simulink model "E_Toothbrush_05"  (Simulink 7.8)
settings: Solver=ode3  StartTime=0.0  StopTime=20  FixedStep=0.001  RelTol=1e-3
undefined symbols (not defined in the file or in its folder): Bar1_length, Bar3_end_xyz, Bar4_length, Body_inertia, Body_mass, Load_torque, Main_gear_r, Motor_gear_r, Motor_speed, Stall_torque
libraries: mblibv1 x31, simulink x1
settings Model: Creator=Harvey  LastModifiedBy=Harvey
settings SimMechanicsCC: VisOnUpdateDiagram=on  VisDuringSimulation=on

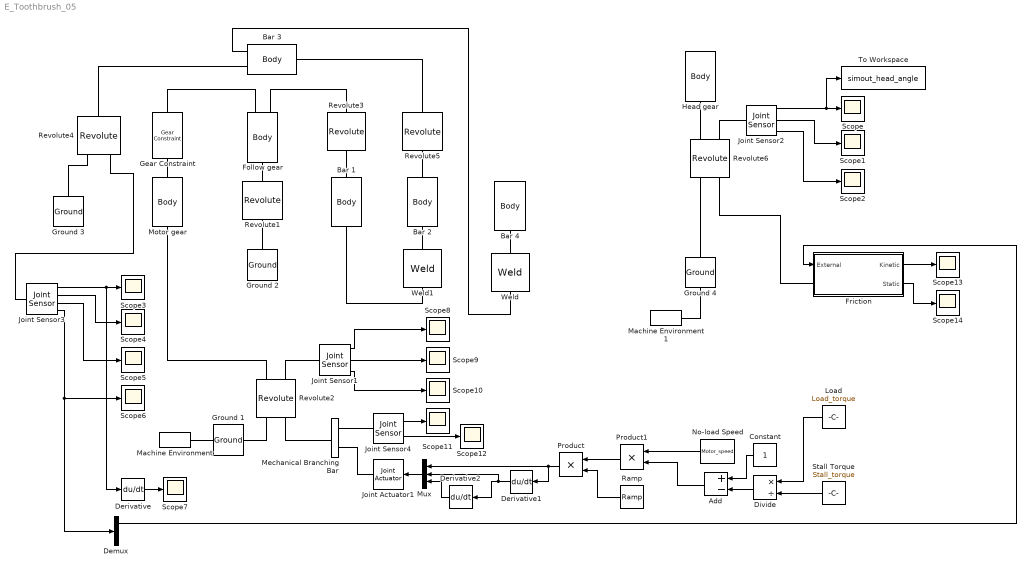
== system E_Toothbrush_05 ==
  Add : Sum  Inputs=+-
  Bar 1 : mblibv1/Bodies/Body  LConnTagsString=CS1  RConnTagsString=CS2  UpdateFromCAD=off  DialogClass=MechanicalBodyBlock  Mass=Body_mass  MassUnits=g  InertiaUnits=g*cm^2  Inertia=Body_inertia  Shape=Cylinder  ShapeDims=[1 1]  ShapeUnits=m  ShapeUse=false  Density=1  DensityUnits=kg/m^3  DensityUse=false  GraphicsMode=MACHINE_DEFAULT  BodyColorSelMode=COLORPALETTE  BodyColor=[0.87059 0.4902 0]  AttachedToCS=CG  CG=Left$CG$[0 0 Bar1_length/2]$CS1$CS1$mm$[0 0 0]$Euler X-Y-Z$deg$WORLD$false$none  WorkingFrames=Left$CS1$[0 0 0]$Adjoining$Adjoining$mm$[0 0 0]$Euler X-Y-Z$deg$WORLD$true$none#Right$CS2$[0 0 Bar1_length]$CS1$CS1$mm$[0 0 0]$Euler X-Y-Z$deg$WORLD$true$none  CGPos=[0 0 Bar1_length/2]  CGRot=[0 0 0]  CS0Pos=[]  CS0Rot=[]  CS1Pos=[0 0 0]  CS1Rot=[0 0 0]  CS2Pos=[0 0 Bar1_length]  CS2Rot=[0 0 0]  CS3Pos=[]  CS3Rot=[]  CS4Pos=[]  CS4Rot=[]  CS5Pos=[]  CS5Rot=[]  CS6Pos=[]  CS6Rot=[]  CS7Pos=[]  CS7Rot=[]  CS8Pos=[]  CS8Rot=[]  CS9Pos=[]  CS9Rot=[]  CS10Pos=[]  CS10Rot=[]  CS11Pos=[]  CS11Rot=[]  CS12Pos=[]  CS12Rot=[]  CS13Pos=[]  CS13Rot=[]  CS14Pos=[]  CS14Rot=[]  CS15Pos=[]  CS15Rot=[]  CS16Pos=[]  CS16Rot=[]  CS17Pos=[]  CS17Rot=[]  CS18Pos=[]  CS18Rot=[]  CS19Pos=[]  CS19Rot=[]  CS20Pos=[]  CS20Rot=[]
  Bar 2 : mblibv1/Bodies/Body  LConnTagsString=CS1  RConnTagsString=CS2  UpdateFromCAD=off  DialogClass=MechanicalBodyBlock  Mass=Body_mass  MassUnits=g  InertiaUnits=g*cm^2  Inertia=Body_inertia  Shape=Cylinder  ShapeDims=[1 1]  ShapeUnits=m  ShapeUse=false  Density=1  DensityUnits=kg/m^3  DensityUse=false  GraphicsMode=MACHINE_DEFAULT  BodyColorSelMode=COLORPALETTE  BodyColor=[0 0 1]  AttachedToCS=CG  CG=Left$CG$[0 0 0]$CS1$CS1$mm$[0 0 0]$Euler X-Y-Z$deg$WORLD$false$none  WorkingFrames=Left$CS1$[0 0 0]$Adjoining$Adjoining$mm$[0 0 0]$Euler X-Y-Z$deg$WORLD$true$none#Right$CS2$[0 0 0]$Adjoining$Adjoining$mm$[0 0 0]$Euler X-Y-Z$deg$WORLD$true$none  CGPos=[0 0 0]  CGRot=[0 0 0]  CS0Pos=[]  CS0Rot=[]  CS1Pos=[0 0 0]  CS1Rot=[0 0 0]  CS2Pos=[0 0 0]  CS2Rot=[0 0 0]  CS3Pos=[]  CS3Rot=[]  CS4Pos=[]  CS4Rot=[]  CS5Pos=[]  CS5Rot=[]  CS6Pos=[]  CS6Rot=[]  CS7Pos=[]  CS7Rot=[]  CS8Pos=[]  CS8Rot=[]  CS9Pos=[]  CS9Rot=[]  CS10Pos=[]  CS10Rot=[]  CS11Pos=[]  CS11Rot=[]  CS12Pos=[]  CS12Rot=[]  CS13Pos=[]  CS13Rot=[]  CS14Pos=[]  CS14Rot=[]  CS15Pos=[]  CS15Rot=[]  CS16Pos=[]  CS16Rot=[]  CS17Pos=[]  CS17Rot=[]  CS18Pos=[]  CS18Rot=[]  CS19Pos=[]  CS19Rot=[]  CS20Pos=[]  CS20Rot=[]
  Bar 3 : mblibv1/Bodies/Body  LConnTagsString=CS2  RConnTagsString=CS3|CS1  UpdateFromCAD=off  DialogClass=MechanicalBodyBlock  Mass=Body_mass  MassUnits=g  InertiaUnits=g*cm^2  Inertia=Body_inertia  Shape=Cylinder  ShapeDims=[1 1]  ShapeUnits=m  ShapeUse=false  Density=1  DensityUnits=kg/m^3  DensityUse=false  GraphicsMode=MACHINE_DEFAULT  BodyColorSelMode=COLORPALETTE  BodyColor=[0 1 0]  AttachedToCS=CG  CG=Left$CG$Bar3_end_xyz/2$CS1$CS1$mm$[0 0 0]$Euler X-Y-Z$deg$WORLD$false$none  WorkingFrames=Right$CS3$[0 0 0]$CS1$CS1$mm$[0 0 0]$Euler X-Y-Z$deg$WORLD$true$none#Right$CS1$[0 0 0]$Adjoining$Adjoining$mm$[0 0 0]$Euler X-Y-Z$deg$WORLD$true$none#Left$CS2$Bar3_end_xyz$CS1$CS1$mm$[0 0 0]$Euler X-Y-Z$deg$WORLD$true$none  CGPos=Bar3_end_xyz/2  CGRot=[0 0 0]  CS0Pos=[]  CS0Rot=[]  CS1Pos=[0 0 0]  CS1Rot=[0 0 0]  CS2Pos=Bar3_end_xyz  CS2Rot=[0 0 0]  CS3Pos=[0 0 0]  CS3Rot=[0 0 0]  CS4Pos=[]  CS4Rot=[]  CS5Pos=[]  CS5Rot=[]  CS6Pos=[]  CS6Rot=[]  CS7Pos=[]  CS7Rot=[]  CS8Pos=[]  CS8Rot=[]  CS9Pos=[]  CS9Rot=[]  CS10Pos=[]  CS10Rot=[]  CS11Pos=[]  CS11Rot=[]  CS12Pos=[]  CS12Rot=[]  CS13Pos=[]  CS13Rot=[]  CS14Pos=[]  CS14Rot=[]  CS15Pos=[]  CS15Rot=[]  CS16Pos=[]  CS16Rot=[]  CS17Pos=[]  CS17Rot=[]  CS18Pos=[]  CS18Rot=[]  CS19Pos=[]  CS19Rot=[]  CS20Pos=[]  CS20Rot=[]
  Bar 4 : mblibv1/Bodies/Body  LConnTagsString=CS1  RConnTagsString=CS2  UpdateFromCAD=off  DialogClass=MechanicalBodyBlock  Mass=Body_mass  MassUnits=g  InertiaUnits=g*cm^2  Inertia=Body_inertia  Shape=Cylinder  ShapeDims=[1 1]  ShapeUnits=m  ShapeUse=false  Density=1  DensityUnits=kg/m^3  DensityUse=false  GraphicsMode=MACHINE_DEFAULT  BodyColorSelMode=COLORPALETTE  BodyColor=[1 1 0]  AttachedToCS=CG  CG=Left$CG$[0 0 Bar4_length/2]$CS1$CS1$mm$[0 0 0]$Euler X-Y-Z$deg$WORLD$false$none  WorkingFrames=Left$CS1$[0 0 0]$Adjoining$Adjoining$mm$[0 0 0]$Euler X-Y-Z$deg$WORLD$true$none#Right$CS2$[0 0 Bar4_length]$CS1$CS1$mm$[0 0 0]$Euler X-Y-Z$deg$WORLD$true$none  CGPos=[0 0 Bar4_length/2]  CGRot=[0 0 0]  CS0Pos=[]  CS0Rot=[]  CS1Pos=[0 0 0]  CS1Rot=[0 0 0]  CS2Pos=[0 0 Bar4_length]  CS2Rot=[0 0 0]  CS3Pos=[]  CS3Rot=[]  CS4Pos=[]  CS4Rot=[]  CS5Pos=[]  CS5Rot=[]  CS6Pos=[]  CS6Rot=[]  CS7Pos=[]  CS7Rot=[]  CS8Pos=[]  CS8Rot=[]  CS9Pos=[]  CS9Rot=[]  CS10Pos=[]  CS10Rot=[]  CS11Pos=[]  CS11Rot=[]  CS12Pos=[]  CS12Rot=[]  CS13Pos=[]  CS13Rot=[]  CS14Pos=[]  CS14Rot=[]  CS15Pos=[]  CS15Rot=[]  CS16Pos=[]  CS16Rot=[]  CS17Pos=[]  CS17Rot=[]  CS18Pos=[]  CS18Rot=[]  CS19Pos=[]  CS19Rot=[]  CS20Pos=[]  CS20Rot=[]
  Constant : Constant
  Demux : Demux  Outputs=3
  Derivative : Derivative
  Derivative1 : Derivative
  Derivative2 : Derivative
  Divide : Product  Inputs=*/
  Follow gear : mblibv1/Bodies/Body  LConnTagsString=CS1  RConnTagsString=CS2|CS3  UpdateFromCAD=off  DialogClass=MechanicalBodyBlock  Mass=Body_mass  MassUnits=g  InertiaUnits=g*cm^2  Inertia=Body_inertia  Shape=Cylinder  ShapeDims=[1 1]  ShapeUnits=m  ShapeUse=false  Density=1  DensityUnits=kg/m^3  DensityUse=false  GraphicsMode=MACHINE_DEFAULT  BodyColorSelMode=COLORPALETTE  BodyColor=[1 0.6 0.78431]  AttachedToCS=CG  CG=Left$CG$[0 0 0]$CS1$CS1$mm$[0 0 0]$Euler X-Y-Z$deg$WORLD$false$none  WorkingFrames=Left$CS1$[0 0 0]$Adjoining$Adjoining$mm$[0 0 0]$Euler X-Y-Z$deg$WORLD$true$none#Right$CS2$[0 0 0]$CS1$CS1$mm$[0 0 0]$Euler X-Y-Z$deg$WORLD$true$none#Right$CS3$Bar1_start_xyz$World$World$mm$[0 0 0]$Euler X-Y-Z$deg$WORLD$true$none  CGPos=[0 0 0]  CGRot=[0 0 0]  CS0Pos=[]  CS0Rot=[]  CS1Pos=[0 0 0]  CS1Rot=[0 0 0]  CS2Pos=[0 0 0]  CS2Rot=[0 0 0]  CS3Pos=Bar1_start_xyz  CS3Rot=[0 0 0]  CS4Pos=[]  CS4Rot=[]  CS5Pos=[]  CS5Rot=[]  CS6Pos=[]  CS6Rot=[]  CS7Pos=[]  CS7Rot=[]  CS8Pos=[]  CS8Rot=[]  CS9Pos=[]  CS9Rot=[]  CS10Pos=[]  CS10Rot=[]  CS11Pos=[]  CS11Rot=[]  CS12Pos=[]  CS12Rot=[]  CS13Pos=[]  CS13Rot=[]  CS14Pos=[]  CS14Rot=[]  CS15Pos=[]  CS15Rot=[]  CS16Pos=[]  CS16Rot=[]  CS17Pos=[]  CS17Rot=[]  CS18Pos=[]  CS18Rot=[]  CS19Pos=[]  CS19Rot=[]  CS20Pos=[]  CS20Rot=[]
  Friction : Subsystem
  Gear Constraint : mblibv1/Constraints &  Drivers/Gear Constraint  LConnTagsString=__newl0  RConnTagsString=__newr0  UpdateFromCAD=off  DialogClass=GearConstraint  NumSAPorts=0  BaseRadius=Motor_gear_r  BaseRadiusUnits=mm  FollowerRadius=Main_gear_r  FollowerRadiusUnits=mm
  Ground 1 : mblibv1/Bodies/Ground  UpdateFromCAD=off  LeftPortType=env  RightPortType=workingframe  PhysicalDomain=Mechanical  DialogClass=GroundBlock  CoordPosition=[0 0 0]  CoordPositionUnits=mm  StateVectorMgrId=2  MachineId=[1 1]  ShowEnvPort=on
  Ground 2 : mblibv1/Bodies/Ground  UpdateFromCAD=off  LeftPortType=env  RightPortType=workingframe  PhysicalDomain=Mechanical  DialogClass=GroundBlock  CoordPosition=[Motor_gear_r+Main_gear_r 0 0]  CoordPositionUnits=mm  StateVectorMgrId=-1  MachineId=[0 0]  ShowEnvPort=off
  Ground 3 : mblibv1/Bodies/Ground  UpdateFromCAD=off  LeftPortType=env  RightPortType=workingframe  PhysicalDomain=Mechanical  DialogClass=GroundBlock  CoordPosition=[0 0 Bar1_length]  CoordPositionUnits=mm  StateVectorMgrId=-1  MachineId=[0 0]  ShowEnvPort=off
  Ground 4 : mblibv1/Bodies/Ground  UpdateFromCAD=off  LeftPortType=env  RightPortType=workingframe  PhysicalDomain=Mechanical  DialogClass=GroundBlock  CoordPosition=Head_xyz  CoordPositionUnits=mm  StateVectorMgrId=3  MachineId=[1 0]  ShowEnvPort=on
  Head gear : mblibv1/Bodies/Body  LConnTagsString=CS1  RConnTagsString=CS2  UpdateFromCAD=off  DialogClass=MechanicalBodyBlock  Mass=1  MassUnits=g  InertiaUnits=g*cm^2  Inertia=Body_inertia  Shape=Cylinder  ShapeDims=[1 1]  ShapeUnits=m  ShapeUse=false  Density=1  DensityUnits=kg/m^3  DensityUse=false  GraphicsMode=MACHINE_DEFAULT  BodyColorSelMode=COLORPALETTE  BodyColor=[0.47843 0.062745 0.89412]  AttachedToCS=CG  CG=Left$CG$[0 0 0]$CS1$CS1$mm$[0 0 0]$Euler X-Y-Z$deg$CS1$false$none  WorkingFrames=Left$CS1$[0 0 0]$Adjoining$Adjoining$mm$[0 0 0]$Euler X-Y-Z$deg$World$true$none#Right$CS2$[0 5 0]$CS1$CS1$mm$[0 0 0]$Euler X-Y-Z$deg$CS1$true$none#Right$CS3$[0 -5 0]$CS1$CS1$mm$[0 0 0]$Euler X-Y-Z$deg$CS1$false$none  CGPos=[0 0 0]  CGRot=[0 0 0]  CS0Pos=[]  CS0Rot=[]  CS1Pos=[0 0 0]  CS1Rot=[0 0 0]  CS2Pos=[0 5 0]  CS2Rot=[0 0 0]  CS3Pos=[0 -5 0]  CS3Rot=[0 0 0]  CS4Pos=[]  CS4Rot=[]  CS5Pos=[]  CS5Rot=[]  CS6Pos=[]  CS6Rot=[]  CS7Pos=[]  CS7Rot=[]  CS8Pos=[]  CS8Rot=[]  CS9Pos=[]  CS9Rot=[]  CS10Pos=[]  CS10Rot=[]  CS11Pos=[]  CS11Rot=[]  CS12Pos=[]  CS12Rot=[]  CS13Pos=[]  CS13Rot=[]  CS14Pos=[]  CS14Rot=[]  CS15Pos=[]  CS15Rot=[]  CS16Pos=[]  CS16Rot=[]  CS17Pos=[]  CS17Rot=[]  CS18Pos=[]  CS18Rot=[]  CS19Pos=[]  CS19Rot=[]  CS20Pos=[]  CS20Rot=[]
  Joint Actuator1 : mblibv1/Sensors &  Actuators/Joint Actuator  UpdateFromCAD=off  PhysicalDomain=Mechanical  PortType=blob  ActuationStyle=Motion  AngleUnits=deg  ArcVelocityUnits=rpm  ArcAccelerationUnits=deg/s^2  CoordPositionUnits=m  VelocityUnits=m/s  AccelerationUnits=m/s^2  ForceUnits=N  TorqueUnits=mN*m  ActiveIO=on  Width=3  DialogClass=MechanicalActuatorBlock  Primitive=R1  ReferenceFrame=Absolute (World)
  Joint Sensor1 : mblibv1/Sensors &  Actuators/Joint Sensor  UpdateFromCAD=off  PhysicalDomain=Mechanical  PortType=blob  Muxed=off  Pose=off  Angle=on  AngleUnits=deg  ArcVelocity=on  ArcVelocityUnits=rpm  ArcAcceleration=off  ArcAccelerationUnits=deg/s^2  CoordPosition=on  CoordPositionUnits=m  Velocity=off  VelocityUnits=m/s  Acceleration=off  AccelerationUnits=m/s^2  Quaternion=on  QuaternionDT=off  QuaternionDDT=off  QuaternionUnits=off  OutputVector=[1]  ActiveIO=on  Width=3  DialogClass=MechanicalSensorBlock  Primitive=R1  Force=off  ForceUnits=N  Torque=on  TorqueUnits=N*m  ReferenceFrame=Absolute (World)  ReactionSensedSide=Follower  ReactionReferenceFrame=Local (Body CS)  ReactionForce=off  ReactionForceUnits=N  ReactionMoment=off  ReactionMomentUnits=N*m
  Joint Sensor2 : mblibv1/Sensors &  Actuators/Joint Sensor  UpdateFromCAD=off  PhysicalDomain=Mechanical  PortType=blob  Muxed=off  Pose=off  Angle=on  AngleUnits=deg  ArcVelocity=on  ArcVelocityUnits=rpm  ArcAcceleration=off  ArcAccelerationUnits=deg/s^2  CoordPosition=on  CoordPositionUnits=m  Velocity=off  VelocityUnits=m/s  Acceleration=off  AccelerationUnits=m/s^2  Quaternion=on  QuaternionDT=off  QuaternionDDT=off  QuaternionUnits=off  OutputVector=[1]  ActiveIO=on  Width=5  DialogClass=MechanicalSensorBlock  Primitive=R1  Force=off  ForceUnits=N  Torque=off  TorqueUnits=N*m  ReferenceFrame=Absolute (World)  ReactionSensedSide=Base  ReactionReferenceFrame=Absolute (World)  ReactionForce=off  ReactionForceUnits=N  ReactionMoment=on  ReactionMomentUnits=N*m
  Joint Sensor3 : mblibv1/Sensors &  Actuators/Joint Sensor  UpdateFromCAD=off  PhysicalDomain=Mechanical  PortType=blob  Muxed=off  Pose=off  Angle=on  AngleUnits=deg  ArcVelocity=on  ArcVelocityUnits=rpm  ArcAcceleration=on  ArcAccelerationUnits=deg/s^2  CoordPosition=on  CoordPositionUnits=m  Velocity=off  VelocityUnits=m/s  Acceleration=off  AccelerationUnits=m/s^2  Quaternion=on  QuaternionDT=off  QuaternionDDT=off  QuaternionUnits=off  OutputVector=[1]  ActiveIO=on  Width=6  DialogClass=MechanicalSensorBlock  Primitive=R1  Force=off  ForceUnits=N  Torque=off  TorqueUnits=N*m  ReferenceFrame=Absolute (World)  ReactionSensedSide=Follower  ReactionReferenceFrame=Absolute (World)  ReactionForce=off  ReactionForceUnits=N  ReactionMoment=on  ReactionMomentUnits=N*m
  Joint Sensor4 : mblibv1/Sensors &  Actuators/Joint Sensor  UpdateFromCAD=off  PhysicalDomain=Mechanical  PortType=blob  Muxed=off  Pose=off  Angle=on  AngleUnits=deg  ArcVelocity=on  ArcVelocityUnits=rpm  ArcAcceleration=off  ArcAccelerationUnits=deg/s^2  CoordPosition=on  CoordPositionUnits=m  Velocity=off  VelocityUnits=m/s  Acceleration=off  AccelerationUnits=m/s^2  Quaternion=on  QuaternionDT=off  QuaternionDDT=off  QuaternionUnits=off  OutputVector=[1]  ActiveIO=on  Width=2  DialogClass=MechanicalSensorBlock  Primitive=R1  Force=off  ForceUnits=N  Torque=off  TorqueUnits=N*m  ReferenceFrame=Absolute (World)  ReactionSensedSide=Base  ReactionReferenceFrame=Absolute (World)  ReactionForce=off  ReactionForceUnits=N  ReactionMoment=off  ReactionMomentUnits=N*m
  Load : Constant  Value=Load_torque
  Machine Environment : mblibv1/Bodies/Machine Environment  PortType=env  PhysicalDomain=Mechanical  DialogTemplateClass=MECH.MachineEnvironment  SyncWhenCopied=off  Gravity=[0 0 -9.81]  GravityUnits=m/s^2  GravityAsSignal=off  Dimensionality=3D Only  AnalysisType=Forward dynamics  LinearAssemblyTolerance=1e-3  LinearAssemblyToleranceUnits=m  AngularAssemblyTolerance=1e-3  AngularAssemblyToleranceUnits=rad  ConstraintSolverType=Stabilizing  ConstraintRelTolerance=1e-4  ConstraintAbsTolerance=1e-4  UseRobustSingularityHandling=off  RedundancyAnalysisToleranceType=Automatically select tolerance  RedundancyAnalysisTolerance=1e-14  StatePerturbationType=Fixed  PerturbationSize=1e-5  VisualizeMachine=on  BodyVisualizationType=Use model default body geometries  BodyColorSelMode=Use model default  DefaultBodyColor=[1 0 0]
  Machine Environment1 : mblibv1/Bodies/Machine Environment  PortType=env  PhysicalDomain=Mechanical  DialogTemplateClass=MECH.MachineEnvironment  SyncWhenCopied=off  Gravity=[0 0 -9.81]  GravityUnits=m/s^2  GravityAsSignal=off  Dimensionality=3D Only  AnalysisType=Forward dynamics  LinearAssemblyTolerance=1e-3  LinearAssemblyToleranceUnits=m  AngularAssemblyTolerance=1e-3  AngularAssemblyToleranceUnits=rad  ConstraintSolverType=Stabilizing  ConstraintRelTolerance=1e-4  ConstraintAbsTolerance=1e-4  UseRobustSingularityHandling=off  RedundancyAnalysisToleranceType=Automatically select tolerance  RedundancyAnalysisTolerance=1e-14  StatePerturbationType=Fixed  PerturbationSize=1e-5  VisualizeMachine=on  BodyVisualizationType=Use model default body geometries  BodyColorSelMode=Use model default  DefaultBodyColor=[1 0 0]
  Mechanical Branching Bar : mblibv1/Utilities/Mechanical Branching Bar  LConnTagsString=_newl0  RConnTagsString=__newr0|SA2  UpdateFromCAD=off  DialogClass=MechanicalBranchingBarBlock  NumSAPorts=2
  Motor gear : mblibv1/Bodies/Body  LConnTagsString=CS1  RConnTagsString=CS2  UpdateFromCAD=off  DialogClass=MechanicalBodyBlock  Mass=Body_mass  MassUnits=g  InertiaUnits=g*cm^2  Inertia=Body_inertia  Shape=Cylinder  ShapeDims=[1 1]  ShapeUnits=m  ShapeUse=false  Density=1  DensityUnits=kg/m^3  DensityUse=false  GraphicsMode=MACHINE_DEFAULT  BodyColorSelMode=COLORPALETTE  BodyColor=[0 1 1]  AttachedToCS=CG  CG=Left$CG$[0 0 0]$CS1$CS1$mm$[0 0 0]$Euler X-Y-Z$deg$WORLD$false$none  WorkingFrames=Left$CS3$[Motor_gear_r 0 0]$CS1$CS1$mm$[0 0 0]$Euler X-Y-Z$deg$WORLD$false$none#Left$CS1$[0 0 0]$Adjoining$Adjoining$mm$[0 0 0]$Euler X-Y-Z$deg$WORLD$true$none#Right$CS2$[0 0 0]$CS1$CS1$mm$[0 0 0]$Euler X-Y-Z$deg$WORLD$true$none  CGPos=[0 0 0]  CGRot=[0 0 0]  CS0Pos=[]  CS0Rot=[]  CS1Pos=[0 0 0]  CS1Rot=[0 0 0]  CS2Pos=[0 0 0]  CS2Rot=[0 0 0]  CS3Pos=[Motor_gear_r 0 0]  CS3Rot=[0 0 0]  CS4Pos=[]  CS4Rot=[]  CS5Pos=[]  CS5Rot=[]  CS6Pos=[]  CS6Rot=[]  CS7Pos=[]  CS7Rot=[]  CS8Pos=[]  CS8Rot=[]  CS9Pos=[]  CS9Rot=[]  CS10Pos=[]  CS10Rot=[]  CS11Pos=[]  CS11Rot=[]  CS12Pos=[]  CS12Rot=[]  CS13Pos=[]  CS13Rot=[]  CS14Pos=[]  CS14Rot=[]  CS15Pos=[]  CS15Rot=[]  CS16Pos=[]  CS16Rot=[]  CS17Pos=[]  CS17Rot=[]  CS18Pos=[]  CS18Rot=[]  CS19Pos=[]  CS19Rot=[]  CS20Pos=[]  CS20Rot=[]
  Mux : Mux  Inputs=3
  No-load Speed : Constant  Value=Motor_speed
  Product : Product  RndMeth=Zero
  Product1 : Product  RndMeth=Zero
  Ramp : simulink/Sources/Ramp  slope=1  start=0  X0=0
  Revolute1 : mblibv1/Joints/Revolute  LConnTagsString=__newl0  RConnTagsString=__newr0  UpdateFromCAD=on  NumSAPorts=0  CutJoint=off  MarkAsCut=off  Primitives=prismatic  PrimitiveProps=R1$World$[0 0 1]$revolute  DialogClass=JointBlock  R1Axis=[0 0 1]
  Revolute2 : mblibv1/Joints/Revolute  LConnTagsString=__newl0|SA1  RConnTagsString=__newr0|SA1  UpdateFromCAD=on  NumSAPorts=2  CutJoint=off  MarkAsCut=off  Primitives=prismatic  PrimitiveProps=R1$World$[0 0 1]$revolute  DialogClass=JointBlock  R1Axis=[0 0 1]
  Revolute3 : mblibv1/Joints/Revolute  LConnTagsString=__newl0  RConnTagsString=__newr0  UpdateFromCAD=on  NumSAPorts=0  CutJoint=off  MarkAsCut=off  Primitives=prismatic  PrimitiveProps=R1$World$[0 0 1]$revolute  DialogClass=JointBlock  R1Axis=[0 0 1]
  Revolute4 : mblibv1/Joints/Revolute  LConnTagsString=__newl0|SA1  RConnTagsString=__newr0  UpdateFromCAD=on  NumSAPorts=1  CutJoint=off  MarkAsCut=off  Primitives=prismatic  PrimitiveProps=R1$World$[0 0 1]$revolute  DialogClass=JointBlock  R1Axis=[0 0 1]
  Revolute5 : mblibv1/Joints/Revolute  LConnTagsString=__newl0  RConnTagsString=__newr0  UpdateFromCAD=on  NumSAPorts=0  CutJoint=off  MarkAsCut=off  Primitives=prismatic  PrimitiveProps=R1$World$[0 0 1]$revolute  DialogClass=JointBlock  R1Axis=[0 0 1]
  Revolute6 : mblibv1/Joints/Revolute  LConnTagsString=__newl0|SA1  RConnTagsString=__newr0|SA1  UpdateFromCAD=on  NumSAPorts=2  CutJoint=off  MarkAsCut=off  Primitives=prismatic  PrimitiveProps=R1$World$Head_direction$revolute  DialogClass=JointBlock  R1Axis=Head_direction
  Scope{,1..14} (15 alike) : Scope
      Scope settings: TimeRange=0.003326971569240389  YMin=32.3459  YMax=35.7507  SaveName=ScopeData3
      Scope1 settings: YMin=0  YMax=22
      Scope10 settings: YMin=0  YMax=22  SaveName=ScopeData4
      Scope11 settings: TimeRange=1  YMin=-4  YMax=3.5  SaveName=ScopeData13
      Scope12 settings: TimeRange=1  YMin=-4  YMax=3.5  SaveName=ScopeData14
      Scope13 settings: TimeRange=1  YMin=-4  YMax=3.5  SaveName=ScopeData2
      Scope14 settings: TimeRange=1  YMin=-4  YMax=3.5  SaveName=ScopeData15
      Scope2 settings: YMin=0  YMax=22  SaveName=ScopeData7
      Scope3 settings: TimeRange=5  YMin=75  YMax=105  SaveName=ScopeData8
      Scope4 settings: YMin=0  YMax=22  SaveName=ScopeData9
      Scope5 settings: YMin=0  YMax=22  SaveName=ScopeData10
      Scope6 settings: YMin=0  YMax=22  SaveName=ScopeData11
      Scope7 settings: YMin=-600  YMax=700  SaveName=ScopeData12
      Scope8 settings: TimeRange=5  YMin=75  YMax=105  SaveName=ScopeData5
      Scope9 settings: YMin=16000  YMax=27500  SaveName=ScopeData6
  Stall Torque : Constant  Value=Stall_torque
  To Workspace : ToWorkspace  VariableName=simout_head_angle  SampleTime=-1  SaveFormat=Array
  Weld : mblibv1/Joints/Weld  LConnTagsString=__newl0  RConnTagsString=__newr0  UpdateFromCAD=off  NumSAPorts=0  CutJoint=off  MarkAsCut=off  Primitives=weld  PrimitiveProps=W$WORLD$[0 0 0]$weld  DialogClass=JointBlock  WAxis=[0 0 0]
  Weld1 : mblibv1/Joints/Weld  LConnTagsString=__newl0  RConnTagsString=__newr0  UpdateFromCAD=off  NumSAPorts=0  CutJoint=off  MarkAsCut=off  Primitives=weld  PrimitiveProps=W$WORLD$[0 0 0]$weld  DialogClass=JointBlock  WAxis=[0 0 0]
  wires:
  Joint Sensor1/2 -> Scope9/1
  Joint Sensor1/3 -> Scope10/1
  Joint Sensor1/1 -> Scope8/1
  Joint Sensor3/2 -> Scope4/1
  Joint Sensor3/3 -> Scope5/1
  Joint Sensor3/1 -> Scope3/1, Derivative/1
  Joint Sensor2/1 -> Scope/1, To Workspace/1
  Joint Sensor2/2 -> Scope1/1
  Joint Sensor2/3 -> Scope2/1
  Joint Sensor3/4 -> Scope6/1, Demux/1
  Derivative/1 -> Scope7/1
  Joint Sensor4/1 -> Scope11/1
  Derivative1/1 -> Mux/2, Derivative2/1
  Derivative2/1 -> Mux/3
  Joint Sensor4/2 -> Scope12/1
  Mux/1 -> Joint Actuator1/1
  Product/1 -> Mux/1, Derivative1/1
  Ramp/1 -> Product/2
  Product1/1 -> Product/1
  No-load Speed/1 -> Product1/1
  Stall Torque/1 -> Divide/2
  Divide/1 -> Add/2
  Constant/1 -> Add/1
  Add/1 -> Product1/2
  Load/1 -> Divide/1
  Demux/1 -> Friction/1(External)
  Friction/1(Kinetic) -> Scope13/1
  Friction/2(Static) -> Scope14/1
  connections:
  Machine Environment/RConn1 -- Ground 1/LConn1
  Ground 1/RConn1 -- Revolute2/LConn1
  Revolute2/RConn1 -- Motor gear/LConn1
  Motor gear/RConn1 -- Gear Constraint/LConn1
  Ground 2/RConn1 -- Revolute1/LConn1
  Revolute1/RConn1 -- Follow gear/LConn1
  Gear Constraint/RConn1 -- Follow gear/RConn1
  Bar 2/RConn1 -- Revolute5/LConn1
  Bar 3/LConn1 -- Revolute5/RConn1
  Follow gear/RConn2 -- Revolute3/LConn1
  Revolute3/RConn1 -- Bar 1/LConn1
  Bar 2/LConn1 -- Weld1/RConn1
  Weld1/LConn1 -- Bar 1/RConn1
  Revolute4/LConn1 -- Ground 3/RConn1
  Bar 3/RConn2 -- Revolute4/RConn1
  Joint Sensor1/LConn1 -- Revolute2/RConn2
  Revolute4/LConn2 -- Joint Sensor3/LConn1
  Bar 4/LConn1 -- Weld/RConn1
  Weld/LConn1 -- Bar 3/RConn1
  Joint Sensor2/LConn1 -- Revolute6/RConn2
  Revolute6/RConn1 -- Head gear/LConn1
  Revolute6/LConn1 -- Ground 4/RConn1
  Friction/LConn1 -- Revolute6/LConn2
  Joint Actuator1/RConn1 -- Mechanical Branching Bar/RConn2
  Mechanical Branching Bar/RConn1 -- Joint Sensor4/LConn1
  Mechanical Branching Bar/LConn1 -- Revolute2/LConn2
  Machine Environment1/RConn1 -- Ground 4/LConn1

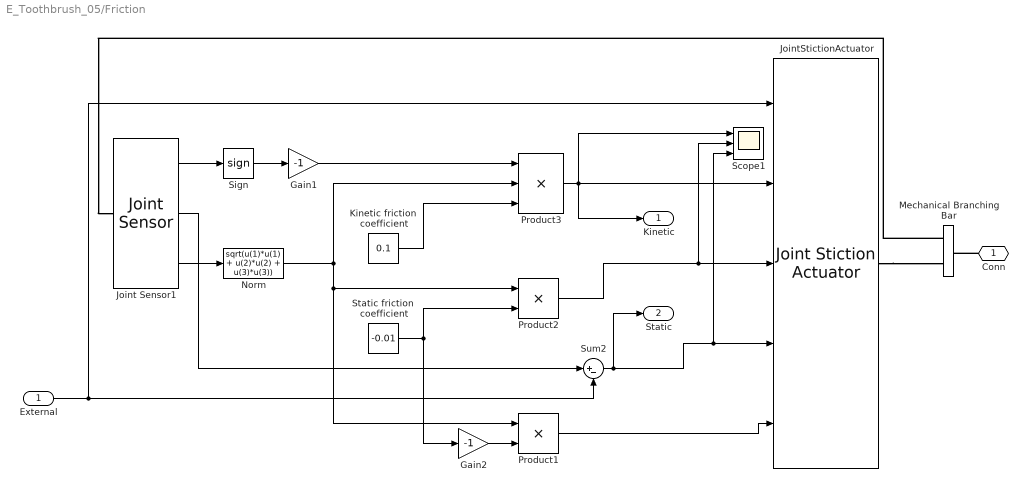
== system E_Toothbrush_05/Friction ==
  External : Inport
  Gain1 : Gain  Gain=-1  SaturateOnIntegerOverflow=on  OutDataTypeStr=Inherit: Same as input  ParamDataTypeStr=Inherit: Same as input
  Gain2 : Gain  Gain=-1  SaturateOnIntegerOverflow=on  OutDataTypeStr=Inherit: Same as input  ParamDataTypeStr=Inherit: Same as input
  Joint Sensor1 : mblibv1/Sensors &  Actuators/Joint Sensor  UpdateFromCAD=off  PhysicalDomain=Mechanical  PortType=blob  Muxed=off  Pose=off  Angle=off  AngleUnits=deg  ArcVelocity=on  ArcVelocityUnits=deg/s  ArcAcceleration=off  ArcAccelerationUnits=deg/s^2  CoordPosition=on  CoordPositionUnits=m  Velocity=off  VelocityUnits=m/s  Acceleration=off  AccelerationUnits=m/s^2  Quaternion=on  QuaternionDT=off  QuaternionDDT=off  QuaternionUnits=off  OutputVector=[1]  ActiveIO=on  Width=5  DialogClass=MechanicalSensorBlock  Primitive=R1  Force=off  ForceUnits=N  Torque=on  TorqueUnits=mN*m  ReferenceFrame=Absolute (World)  ReactionSensedSide=Follower  ReactionReferenceFrame=Local (Body CS)  ReactionForce=on  ReactionForceUnits=mN  ReactionMoment=off  ReactionMomentUnits=mN*m
  JointStictionActuator : mblibv1/Sensors &  Actuators/Joint Stiction Actuator  UpdateFromCAD=off  PhysicalDomain=Mechanical  PortType=blob  ActuationStyle=Force  AngleUnits=deg  ArcVelocityUnits=deg/s  ArcAccelerationUnits=deg/s^2  CoordPositionUnits=m  VelocityUnits=m/s  AccelerationUnits=m/s^2  ForceUnits=N  TorqueUnits=N-m  ActiveIO=on  Width=5  DialogClass=EventActuatorBlock  Primitive=R1  FrictionalForceUnits=N  ExternalForceUnits=N  FrictionalTorqueUnits=mN*m  ExternalTorqueUnits=mN*m  LockingTolerance=1e-2
      link override MSB_SIGNAL_BLOCK: GotoTag=sim_mech_tag6f78254795838dc  TagVisibility=global
  Kinetic friction  coefficient : Constant  Value=0.1
  Mechanical Branching Bar : mblibv1/Utilities/Mechanical Branching Bar  LConnTagsString=_newl0  RConnTagsString=__newr0|SA2  UpdateFromCAD=off  DialogClass=MechanicalBranchingBarBlock  NumSAPorts=2
  Norm : Fcn  Expr=sqrt(u(1)*u(1) + u(2)*u(2) + u(3)*u(3))
  Product1 : Product  SaturateOnIntegerOverflow=on  InputSameDT=on  OutDataTypeStr=Inherit: Same as first input
  Product2 : Product  SaturateOnIntegerOverflow=on  InputSameDT=on  OutDataTypeStr=Inherit: Same as first input
  Product3 : Product  Inputs=3  SaturateOnIntegerOverflow=on  InputSameDT=on  OutDataTypeStr=Inherit: Same as first input
  Scope1 : Scope  NumInputPorts=3
      settings: TimeRange=1  YMin=-1~-66.6739~2  YMax=1~-66.6739~2
  Sign : Signum  ZeroCross=off
  "Static friction  coefficient " : Constant  Value=-0.01
  Sum2 : Sum  Inputs=|+-  SaturateOnIntegerOverflow=on  InputSameDT=on  OutDataTypeStr=Inherit: Same as first input
  Conn : PMIOPort  Port=1  Side=Left
  Kinetic : Outport
  Static : Outport  Port=2
  wires:
  Product1/1 -> JointStictionActuator/5
  Sum2/1 -> Scope1/3, JointStictionActuator/4, Static/1
  Product2/1 -> Scope1/2, JointStictionActuator/3
  Product3/1 -> Kinetic/1, JointStictionActuator/2, Scope1/1
  Gain2/1 -> Product1/2
  External/1 -> JointStictionActuator/1, Sum2/2
  Joint Sensor1/2 -> Sum2/1
  "Static friction  coefficient "/1 -> Gain2/1, Product2/2
  Kinetic friction  coefficient/1 -> Product3/3
  Norm/1 -> Product1/1, Product2/1, Product3/2
  Joint Sensor1/3 -> Norm/1
  Gain1/1 -> Product3/1
  Sign/1 -> Gain1/1
  Joint Sensor1/1 -> Sign/1
  connections:
  Mechanical Branching Bar/RConn1 -- Joint Sensor1/LConn1
  JointStictionActuator/RConn1 -- Mechanical Branching Bar/RConn2
  Conn/RConn1 -- Mechanical Branching Bar/LConn1
